simulink model "pid_exSolved"  (R2018b)
settings: Solver=ode45  StartTime=0.0  StopTime=10.0  RelTol=1e-3  EnableMultiTasking=on
PreLoadFcn:
  | Ts = 0.2;
settings Model: Creator=nicholas  LastModifiedBy=Bob-o Swaggins
settings DataIOCC: LimitDataPoints=on  SaveFormat=Array  SignalLoggingName=sigsOut
settings OptimizationCC: ExpressionDepthLimit=2147483647  InitFltsAndDblsToZero=on  LifeSpan=inf
settings DebuggingCC: SaveWithParameterizedLinksMsg=none  UnderspecifiedInitializationDetection=Classic  MergeDetectMultiDrivingBlocksExec=none  SignalResolutionControl=TryResolveAllWithWarning  MultiTaskDSMMsg=warning  MultiTaskCondExecSysMsg=none  ParameterPrecisionLossMsg=none  FcnCallInpInsideContextMsg=warning  AllowSymbolicDim=off  StateNameClashWarn=warning  LibraryContextMissingDiagnostic=none  SFUnexpectedBacktrackingDiag=warning  SFNoUnconditionalDefaultTransitionDiag=warning  SFExecutionAtInitializationDiag=none
settings HardwareCC: ProdBitPerPointer=32  ProdBitPerSizeT=32  ProdBitPerPtrDiffT=32  ProdLargestAtomicFloat=None  ProdIntDivRoundTo=Undefined  ProdEndianess=Unspecified  ProdWordSize=32  ProdHWDeviceType=32-bit Generic  TargetUnknown=on
settings ModelReferenceCC: PropagateSignalLabelsOutOfModel=off
settings SFSimCC: SimUseLocalCustomCode=off
settings RTWCC: RTWUseLocalCustomCode=off
settings CodeAppCC: StateflowObjectComments=on
settings GRTTargetCC: TargetFcnLib=ansi_tfl_tmw.mat  TargetLangStandard=C89/C90 (ANSI)  GeneratePreprocessorConditionals=Disable all  CombineOutputUpdateFcns=off  GRTInterface=on
settings ConfigComp: CovMetricSettings=dw  CovHtmlReporting=on  CovSaveCumulativeToWorkspaceVar=on  CovSaveSingleToWorkspaceVar=on  CovExternalEMLEnable=off  CovSFcnEnable=off

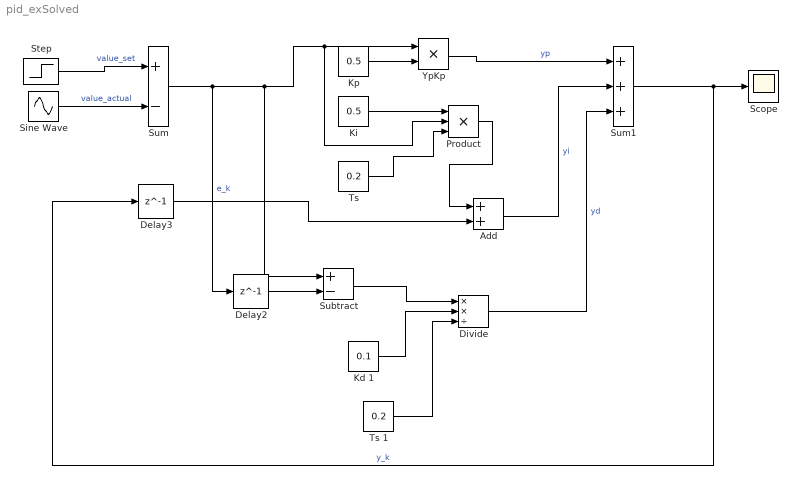
== system pid_exSolved ==
  Add : Sum
  Delay2 : Delay  DelayLength=1  InitialCondition=0
  Delay3 : Delay  DelayLength=1  InitialCondition=0
  Divide : Product  Inputs=**/
  Kd 1 : Constant  Value=0.1
  "Ki " : Constant  Value=0.5
  Kp : Constant  Value=0.5
  Product : Product  Inputs=3
  Scope : Scope
  Sine Wave : Sin  SampleTime=Ts
  Step : Step  SampleTime=Ts
  Subtract : Sum  Inputs=+-
  Sum : Sum  Inputs=+-  SaturateOnIntegerOverflow=on  InputSameDT=on  OutDataTypeStr=Inherit: Same as first input
  Sum1 : Sum  Inputs=+++  SaturateOnIntegerOverflow=on  InputSameDT=on  OutDataTypeStr=Inherit: Same as first input
  "Ts " : Constant  Value=0.2
  Ts 1 : Constant  Value=0.2
  YpKp : Product
  wires:
  Sum1/1 -> Delay3/1, Scope/1  "y_k"
  Step/1 -> Sum/1  "value_set"
  Sine Wave/1 -> Sum/2  "value_actual"
  Sum/1 -> Delay2/1, Subtract/1, Product/2, YpKp/1  "e_k"
  YpKp/1 -> Sum1/1  "yp"
  Kp/1 -> YpKp/2
  "Ki "/1 -> Product/1
  "Ts "/1 -> Product/3
  Product/1 -> Add/1
  Add/1 -> Sum1/2  "yi"
  Subtract/1 -> Divide/1
  Ts 1/1 -> Divide/3
  Kd 1/1 -> Divide/2
  Divide/1 -> Sum1/3  "yd"
  Delay3/1 -> Add/2
  Delay2/1 -> Subtract/2
